simulink library "eulDot"  (R2022a)
settings: Solver=VariableStepAuto  StartTime=0.0  StopTime=10.0  RelTol=1e-3
settings Model: Creator=asiddiq2  LastModifiedBy=lhill8
settings SolverCC: AlgebraicLoopSolver=TrustRegion
settings DebuggingCC: UnconnectedInputMsg=warning  UnconnectedOutputMsg=warning  UnconnectedLineMsg=warning  SFMachineParentedDataDiag=warning  ArithmeticOperatorsInVariantConditions=warning
settings SFSimCC: CustomCodeUndefinedFunction=UseInterfaceOnly

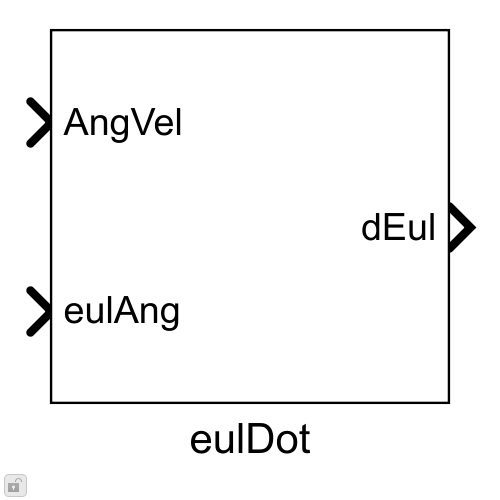
[thumbnail: Simulink's stored preview of the top-level diagram]
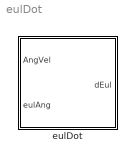
== system eulDot ==
  eulDot : Subsystem

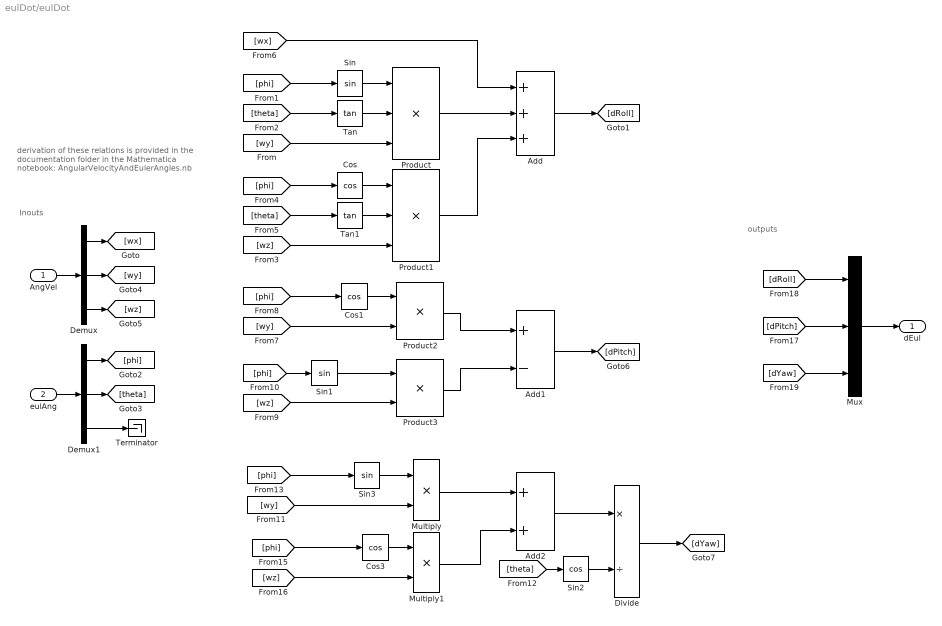
== system eulDot/eulDot ==
  note: derivation of these relations is provided in
      | the documentation folder in the Mathematica
      | notebook: AngularVelocityAndEulerAngles.nb
  note: outputs
  note: Inouts
  AngVel : Inport
  eulAng : Inport  Port=2
  Add : Sum  Inputs=+++
  Add1 : Sum  Inputs=+-
  Add2 : Sum
  Cos : Trigonometry  Operator=cos
  Cos1 : Trigonometry  Operator=cos
  Cos3 : Trigonometry  Operator=cos
  Demux : Demux  Outputs=3
  Demux1 : Demux  Outputs=3
  Divide : Product  Inputs=*/
  Multiply : Product
  Multiply1 : Product
  Mux : Mux  Inputs=3
  Product : Product  Inputs=3
  Product1 : Product  Inputs=3
  Product2 : Product
  Product3 : Product
  Sin : Trigonometry
  Sin1 : Trigonometry
  Sin2 : Trigonometry  Operator=cos
  Sin3 : Trigonometry
  Tan : Trigonometry  Operator=tan
  Tan1 : Trigonometry  Operator=tan
  Terminator : Terminator
  dEul : Outport  VectorParamsAs1DForOutWhenUnconnected=off
  wires:
  Demux1/3 -> Terminator/1
  Sin/1 -> Product/1
  Tan/1 -> Product/2
  [wy] -> Product/3
  [phi] -> Sin/1
  [theta] -> Tan/1
  Cos/1 -> Product1/1
  Tan1/1 -> Product1/2
  [wz] -> Product1/3
  [theta] -> Tan1/1
  [phi] -> Cos/1
  Product/1 -> Add/2
  [wx] -> Add/1
  Product1/1 -> Add/3
  Add/1 -> [dRoll]
  [phi] -> Cos1/1
  Cos1/1 -> Product2/1
  [wy] -> Product2/2
  Sin1/1 -> Product3/1
  [wz] -> Product3/2
  [phi] -> Sin1/1
  Product2/1 -> Add1/1
  Product3/1 -> Add1/2
  [theta] -> Sin2/1
  [phi] -> Sin3/1
  Sin2/1 -> Divide/2
  Sin3/1 -> Multiply/1
  [wy] -> Multiply/2
  [phi] -> Cos3/1
  Cos3/1 -> Multiply1/1
  [wz] -> Multiply1/2
  Multiply/1 -> Add2/1
  Multiply1/1 -> Add2/2
  Demux/1 -> [wx]
  Demux/2 -> [wy]
  Demux/3 -> [wz]
  AngVel/1 -> Demux/1
  eulAng/1 -> Demux1/1
  Demux1/1 -> [phi]
  Demux1/2 -> [theta]
  Add1/1 -> [dPitch]
  Add2/1 -> Divide/1
  [dPitch] -> Mux/2
  [dRoll] -> Mux/1
  [dYaw] -> Mux/3
  Mux/1 -> dEul/1
  Divide/1 -> [dYaw]
